simulink model "greenhouse"  (R2022b)
settings: Solver=ode45  StartTime=0.0  StopTime=168  FixedStep=1  RelTol=1e-3  AbsTol=1e-6
model workspace (MATLAB code in the model file):
  | % load initial conditions and physical properties from file
  | greenhouse_data
values from neighbouring files (symbols this model uses):
  c = 0.000279277778    [greenhouse_data.m]
  cost = 0.12    [greenhouse_data.m]
  M = Volume*densAir    (= 675.28125)    [greenhouse_data.m]
  Mdot = 3600    [greenhouse_data.m]
  Req = RBrick*RPC/(RBrick + RPC)    (= 1.00870802569)    [greenhouse_data.m]
  THeater = 47    [greenhouse_data.m]
  TRefrigerator = 10    [greenhouse_data.m]
libraries: simulink x2
Description:
  | Thermal Model of a House
  | 
  | This demo illustrates how you can use Simulink(R) to create the thermal model of
  | a house. This system models the outdoor environment, the thermal
  | characteristics of the house, and the house heating system.
  | 
  | The sldemo_househeat_data.m file initializes data in the model workspace.
  | To make changes, you can edit the model workspace directly or edit the MATLAB(R) file
  | and re-load the model workspace.
  | 
  | To view the model workspace, select View > Model Explorer
  | from the Simulink editor.
  | 
  | Note: Time is given in units of hours
settings Model: Creator=The MathWorks, Inc.  LastModifiedBy=Usuario
settings SolverCC: AutoScaleAbsTol=off  AlgebraicLoopSolver=TrustRegion
settings DataIOCC: ExternalInput=[]  InitialState=[]  SaveFormat=Array  SaveOutput=off  SaveTime=off  SignalLoggingName=sldemo_househeat_output
settings OptimizationCC: BlockReduction=off  BooleanDataType=off  ExpressionDepthLimit=2147483647  InitFltsAndDblsToZero=on  LifeSpan=inf  BufferReusableBoundary=off
settings DebuggingCC: SaveWithParameterizedLinksMsg=none  UnderspecifiedInitializationDetection=Classic  MergeDetectMultiDrivingBlocksExec=none  SignalResolutionControl=TryResolveAllWithWarning  MultiTaskDSMMsg=warning  MultiTaskCondExecSysMsg=none  IntegerOverflowMsg=none  FcnCallInpInsideContextMsg=warning  UnconnectedInputMsg=warning  UnconnectedOutputMsg=warning  UnconnectedLineMsg=warning  BusObjectLabelMismatch=none  StateNameClashWarn=warning  SFUnexpectedBacktrackingDiag=warning  SFNoUnconditionalDefaultTransitionDiag=warning  SFExecutionAtInitializationDiag=none  SFMachineParentedDataDiag=warning  IntegerSaturationMsg=none  ArithmeticOperatorsInVariantConditions=warning
settings HardwareCC: ProdBitPerPointer=32  ProdBitPerSizeT=32  ProdBitPerPtrDiffT=32  ProdLargestAtomicFloat=None  ProdIntDivRoundTo=Undefined  ProdEndianess=Unspecified  ProdWordSize=32  ProdHWDeviceType=32-bit Generic  TargetUnknown=on
settings ModelReferenceCC: EnableRefExpFcnMdlSchedulingChecks=on  PropagateSignalLabelsOutOfModel=off
settings SFSimCC: SimUseLocalCustomCode=off  CustomCodeUndefinedFunction=UseInterfaceOnly
settings RTWCC: RTWUseLocalCustomCode=off
settings CodeAppCC: StateflowObjectComments=on
settings GRTTargetCC: TargetFcnLib=ansi_tfl_tmw.mat  TargetLangStandard=C89/C90 (ANSI)  CombineOutputUpdateFcns=off  GRTInterface=on
settings ConfigComp: CovMetricSettings=dw  CovSaveCumulativeToWorkspaceVar=on  CovSaveSingleToWorkspaceVar=on  CovExternalEMLEnable=off

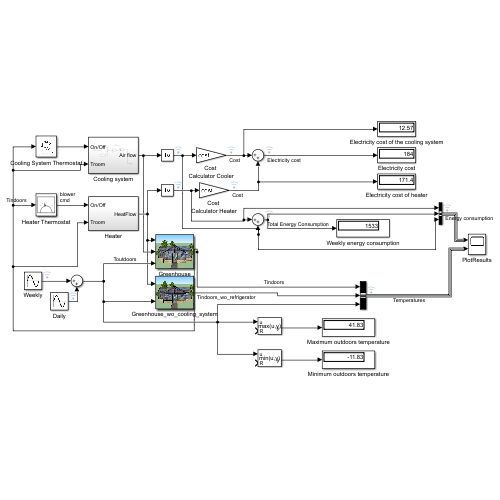
[thumbnail: Simulink's stored preview of the top-level diagram]
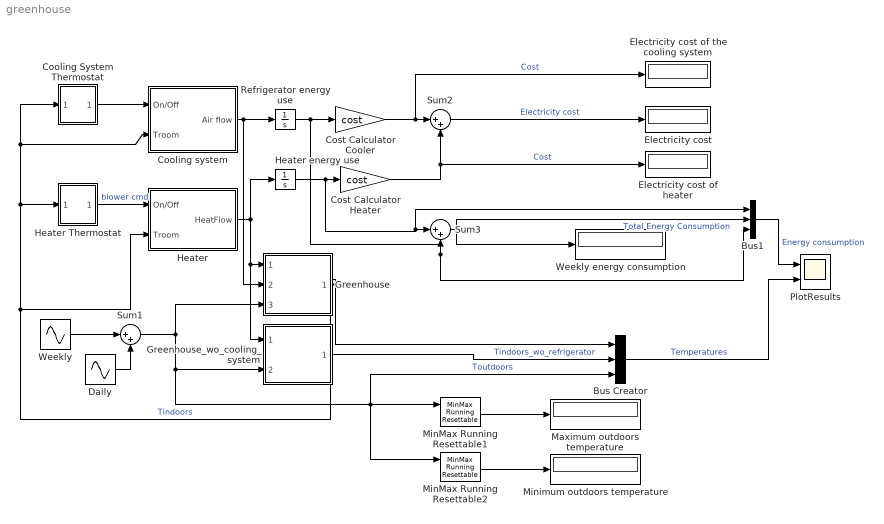
== system greenhouse ==
  Bus Creator : BusCreator  Inputs=3
  Bus1 : BusCreator  Inputs=3
  Cooling System Thermostat : Subsystem
      mask Display: image('$imagefile'); % Use "Edit Image" on toolstrip to change.
  Cooling system : Subsystem
  Cost Calculator Cooler : Gain  Gain=cost  SaturateOnIntegerOverflow=on  OutDataTypeStr=Inherit: Same as input  ParamDataTypeStr=Inherit: Same as input
  Cost Calculator Heater : Gain  Gain=cost  SaturateOnIntegerOverflow=on  OutDataTypeStr=Inherit: Same as input  ParamDataTypeStr=Inherit: Same as input
  Daily : Sin  Amplitude=16  Frequency=2*pi/24  SampleTime=0
  Electricity cost : Display
  Electricity cost of heater : Display
  Electricity cost of the cooling system : Display
  Greenhouse : Subsystem
      mask Display: image('$imagefile'); % Use "Edit Image" on toolstrip to change.
  Greenhouse_wo_cooling_system : Subsystem
      mask Display: image('$imagefile'); % Use "Edit Image" on toolstrip to change.
  Heater : Subsystem
  Heater Thermostat : Subsystem
      mask Display: image(fullfile(matlabroot,'toolbox','simulink','simdemos','simgeneral','images','HouseHeatThermostatPix.svg'))
  Heater energy use : Integrator
  Maximum outdoors temperature : Display
  MinMax Running Resettable1 : simulink/Math Operations/MinMax Running Resettable  Function=max  vinit=30
  MinMax Running Resettable2 : simulink/Math Operations/MinMax Running Resettable  Function=min  vinit=30
  Minimum outdoors temperature : Display
  PlotResults : Scope  NumInputPorts=2
  Refrigerator energy use : Integrator
  Sum1 : Sum  Inputs=|++  InputSameDT=on  SaturateOnIntegerOverflow=on  OutDataTypeStr=Inherit: Same as first input
  Sum2 : Sum  Inputs=|++  InputSameDT=on  SaturateOnIntegerOverflow=on  OutDataTypeStr=Inherit: Same as first input
  Sum3 : Sum  Inputs=|++  InputSameDT=on  SaturateOnIntegerOverflow=on  OutDataTypeStr=Inherit: Same as first input
  Weekly : Sin  Amplitude=12  Bias=15  Frequency=2*pi/168  SampleTime=0
  Weekly energy consumption : Display
  wires:
  Heater energy use/1 -> Bus1/1, Sum3/1, Cost Calculator Heater/1
  Heater Thermostat/1(Blower switch) -> Heater/1(On/Off)  "blower cmd"
  Daily/1 -> Sum1/2
  Sum1/1 -> Greenhouse_wo_cooling_system/2(Outdoor Temp Tout), MinMax Running Resettable1/1, MinMax Running Resettable2/1, Bus Creator/3, Greenhouse/3(Outdoor Temp Tout)  "Toutdoors"
  Weekly/1 -> Sum1/1
  Greenhouse/1(Room Temp Troom) -> Bus Creator/1, Cooling System Thermostat/1(Tindoors), Cooling system/2(Troom), Heater Thermostat/1(Terr), Heater/2(Troom)  "Tindoors"
  Heater/1(HeatFlow) -> Heater energy use/1, Greenhouse_wo_cooling_system/1(Heater QDot In), Greenhouse/1(Heater QDot In)
  Bus Creator/1 -> PlotResults/2  "Temperatures"
  Cooling System Thermostat/1(Out1) -> Cooling system/1(On/Off)
  Cooling system/1(Air flow) -> Greenhouse/2(Refrigerator), Refrigerator energy use/1
  Refrigerator energy use/1 -> Bus1/3, Sum3/2, Cost Calculator Cooler/1
  Cost Calculator Heater/1 -> Electricity cost of heater/1, Sum2/2  "Cost"
  Cost Calculator Cooler/1 -> Electricity cost of the cooling system/1, Sum2/1  "Cost"
  MinMax Running Resettable1/1 -> Maximum outdoors temperature/1
  MinMax Running Resettable2/1 -> Minimum outdoors temperature/1
  Sum2/1 -> Electricity cost/1  "Electricity cost"
  Sum3/1 -> Bus1/2, Weekly energy consumption/1  "Total Energy Consumption"
  Bus1/1 -> PlotResults/1  "Energy consumption"
  Greenhouse_wo_cooling_system/1(Room Temp Troom) -> Bus Creator/2  "Tindoors_wo_refrigerator"

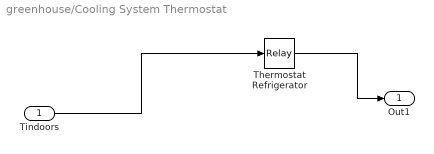
== system greenhouse/Cooling System Thermostat ==
  Tindoors : Inport
  Thermostat Refrigerator : Relay  OnSwitchValue=35  OffSwitchValue=29
  Out1 : Outport
  wires:
  Tindoors/1 -> Thermostat Refrigerator/1
  Thermostat Refrigerator/1 -> Out1/1

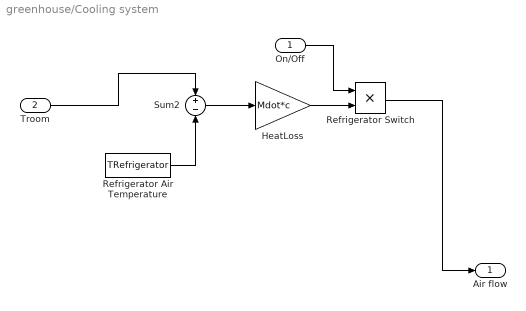
== system greenhouse/Cooling system ==
  On/Off : Inport
  Troom : Inport  Port=2
  HeatLoss : Gain  Gain=Mdot*c
  Refrigerator Air Temperature : Constant  Value=TRefrigerator
  Refrigerator Switch : Product  RndMeth=Zero
  Sum2 : Sum  Inputs=+-
  Air flow : Outport
  wires:
  On/Off/1 -> Refrigerator Switch/1
  Sum2/1 -> HeatLoss/1
  Refrigerator Switch/1 -> Air flow/1
  HeatLoss/1 -> Refrigerator Switch/2
  Refrigerator Air Temperature/1 -> Sum2/2
  Troom/1 -> Sum2/1

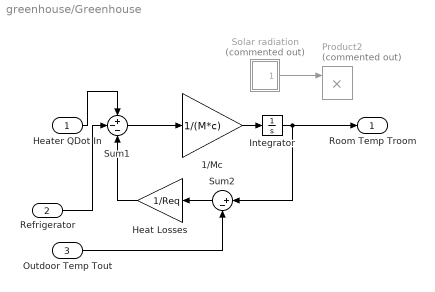
== system greenhouse/Greenhouse ==
  Heater QDot In : Inport
  Refrigerator : Inport  Port=2
  Outdoor Temp Tout : Inport  Port=3
  1/Mc : Gain  Gain=1/(M*c)  SaturateOnIntegerOverflow=on  OutDataTypeStr=Inherit: Same as input  ParamDataTypeStr=Inherit: Same as input
  Heat Losses : Gain  Gain=1/Req  SaturateOnIntegerOverflow=on  OutDataTypeStr=Inherit: Same as input  ParamDataTypeStr=Inherit: Same as input
  Integrator : Integrator  InitialCondition=20
  Product2 : Product  Commented=on
  Solar radiation : Subsystem  Commented=on
      mask Display: image('$imagefile'); % Use "Edit Image" on toolstrip to change.
  Sum1 : Sum  Inputs=+--  InputSameDT=on  SaturateOnIntegerOverflow=on  OutDataTypeStr=Inherit: Same as first input
  Sum2 : Sum  Inputs=|+-  InputSameDT=on  SaturateOnIntegerOverflow=on  OutDataTypeStr=Inherit: Same as first input
  Room Temp Troom : Outport  InitialOutput=0  VectorParamsAs1DForOutWhenUnconnected=off
  wires:
  Outdoor Temp Tout/1 -> Sum2/2
  Heater QDot In/1 -> Sum1/1
  Sum2/1 -> Heat Losses/1
  Heat Losses/1 -> Sum1/3
  Refrigerator/1 -> Sum1/2
  Integrator/1 -> Room Temp Troom/1, Sum2/1
  1/Mc/1 -> Integrator/1
  Sum1/1 -> 1/Mc/1
  Solar radiation/1(Out1) -> Product2/1

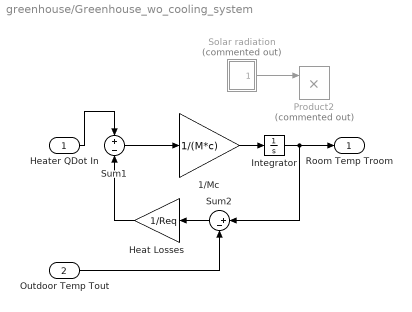
== system greenhouse/Greenhouse_wo_cooling_system ==
  Heater QDot In : Inport
  Outdoor Temp Tout : Inport  Port=2
  1/Mc : Gain  Gain=1/(M*c)  SaturateOnIntegerOverflow=on  OutDataTypeStr=Inherit: Same as input  ParamDataTypeStr=Inherit: Same as input
  Heat Losses : Gain  Gain=1/Req  SaturateOnIntegerOverflow=on  OutDataTypeStr=Inherit: Same as input  ParamDataTypeStr=Inherit: Same as input
  Integrator : Integrator  InitialCondition=20
  Product2 : Product  Commented=on
  Solar radiation : Subsystem  Commented=on
      mask Display: image('$imagefile'); % Use "Edit Image" on toolstrip to change.
  Sum1 : Sum  Inputs=+-  InputSameDT=on  SaturateOnIntegerOverflow=on  OutDataTypeStr=Inherit: Same as first input
  Sum2 : Sum  Inputs=|+-  InputSameDT=on  SaturateOnIntegerOverflow=on  OutDataTypeStr=Inherit: Same as first input
  Room Temp Troom : Outport  InitialOutput=0  VectorParamsAs1DForOutWhenUnconnected=off
  wires:
  Integrator/1 -> Room Temp Troom/1, Sum2/1
  1/Mc/1 -> Integrator/1
  Sum2/1 -> Heat Losses/1
  Sum1/1 -> 1/Mc/1
  Heater QDot In/1 -> Sum1/1
  Outdoor Temp Tout/1 -> Sum2/2
  Heat Losses/1 -> Sum1/2
  Solar radiation/1(Out1) -> Product2/1

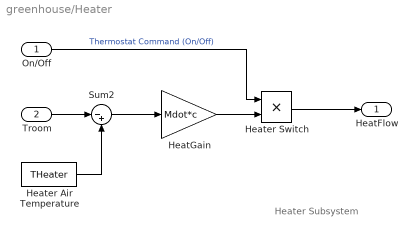
== system greenhouse/Heater ==
  note: Heater Subsystem
  On/Off : Inport
  Troom : Inport  Port=2
  HeatGain : Gain  Gain=Mdot*c
  Heater Air Temperature : Constant  Value=THeater
  Heater Switch : Product  RndMeth=Zero
  Sum2 : Sum  Inputs=|-+
  HeatFlow : Outport  VectorParamsAs1DForOutWhenUnconnected=off
  wires:
  Heater Air Temperature/1 -> Sum2/2
  Troom/1 -> Sum2/1
  Sum2/1 -> HeatGain/1
  On/Off/1 -> Heater Switch/1  "Thermostat Command (On/Off)"
  HeatGain/1 -> Heater Switch/2
  Heater Switch/1 -> HeatFlow/1

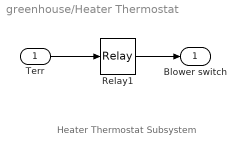
== system greenhouse/Heater Thermostat ==
  note: Heater Thermostat Subsystem
  Terr : Inport
  Relay1 : Relay  OnSwitchValue=23  OffSwitchValue=17  OnOutputValue=0  OffOutputValue=1
  Blower switch : Outport  InitialOutput=0  VectorParamsAs1DForOutWhenUnconnected=off
  wires:
  Terr/1 -> Relay1/1
  Relay1/1 -> Blower switch/1

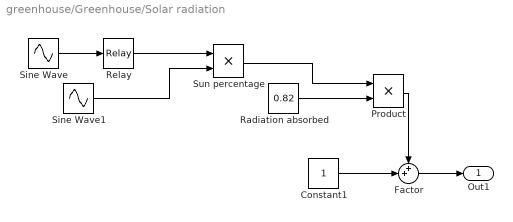
== system greenhouse/Greenhouse/Solar radiation ==
  Constant1 : Constant
  Factor : Sum  Inputs=++|
  "Product " : Product
  Radiation absorbed : Constant  Value=0.82
  Relay : Relay  OnSwitchValue=0.00001  OffSwitchValue=-0.00001
  Sine Wave : Sin  Frequency=2*pi/24  SampleTime=0
  Sine Wave1 : Sin  Frequency=2*pi/24  SampleTime=0
  Sun percentage : Product
  Out1 : Outport
  wires:
  Sine Wave/1 -> Relay/1
  Sun percentage/1 -> "Product "/1
  Relay/1 -> Sun percentage/1
  "Product "/1 -> Factor/1
  Constant1/1 -> Factor/2
  Sine Wave1/1 -> Sun percentage/2
  Radiation absorbed/1 -> "Product "/2
  Factor/1 -> Out1/1

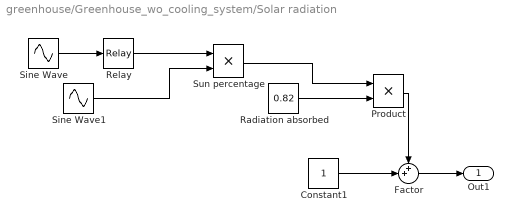
== system greenhouse/Greenhouse_wo_cooling_system/Solar radiation ==
  Constant1 : Constant
  Factor : Sum  Inputs=++|
  "Product " : Product
  Radiation absorbed : Constant  Value=0.82
  Relay : Relay  OnSwitchValue=0.00001  OffSwitchValue=-0.00001
  Sine Wave : Sin  Frequency=2*pi/24  SampleTime=0
  Sine Wave1 : Sin  Frequency=2*pi/24  SampleTime=0
  Sun percentage : Product
  Out1 : Outport
  wires:
  Sine Wave/1 -> Relay/1
  Sun percentage/1 -> "Product "/1
  Relay/1 -> Sun percentage/1
  "Product "/1 -> Factor/1
  Constant1/1 -> Factor/2
  Sine Wave1/1 -> Sun percentage/2
  Radiation absorbed/1 -> "Product "/2
  Factor/1 -> Out1/1
